simulink model "lab5"  (R2022a)
settings: Solver=ode3  StartTime=0.0  StopTime=Stop_time  FixedStep=1e-6  RelTol=1e-5
undefined symbols (not defined in the file): C_dc_filter, gamma, J_s, k_e, k_m, L_a, R_a, Stop_time, T_e_rated, T_e_st, T_Load, T_sw, tau_m, U_s, U_s_rated
libraries: simulink x13, spsMosfetLib x4, spsCurrentMeasurementLib x3, spsVoltageMeasurementLib x3, spsSeriesRLCBranchLib x2, spsControlledVoltageSourceLib x2, spsDiodeLib x2, spsIGBTLib x1, spspowerguiLib x1
settings Model: Creator=PC  LastModifiedBy=81502
settings SolverCC: ZeroCrossControl=DisableAll  AlgebraicLoopSolver=TrustRegion
settings DataIOCC: LimitDataPoints=on  SaveFormat=Array  SignalLoggingSaveFormat=ModelDataLogs  ReturnWorkspaceOutputs=off
settings OptimizationCC: LifeSpan=inf
settings DebuggingCC: UnderspecifiedInitializationDetection=Classic  MergeDetectMultiDrivingBlocksExec=none  SolverPrmCheckMsg=warning  FcnCallInpInsideContextMsg=warning  UnconnectedInputMsg=warning  UnconnectedOutputMsg=warning  UnconnectedLineMsg=warning  SFUnexpectedBacktrackingDiag=warning  SFNoUnconditionalDefaultTransitionDiag=warning  SFExecutionAtInitializationDiag=none  SFMachineParentedDataDiag=warning  ArithmeticOperatorsInVariantConditions=warning
settings HardwareCC: ProdBitPerPointer=32  ProdBitPerSizeT=32  ProdBitPerPtrDiffT=32  ProdLargestAtomicFloat=None  ProdIntDivRoundTo=Undefined  ProdEndianess=Unspecified  ProdWordSize=32  ProdHWDeviceType=32-bit Generic
settings ModelReferenceCC: PropagateSignalLabelsOutOfModel=off
settings SFSimCC: SimUseLocalCustomCode=off  CustomCodeUndefinedFunction=UseInterfaceOnly
settings RTWCC: RTWUseLocalCustomCode=off  DLArmComputeVersion=19.05
settings CodeAppCC: StateflowObjectComments=on
settings GRTTargetCC: TargetLangStandard=C89/C90 (ANSI)  CombineOutputUpdateFcns=off  GRTInterface=on
settings ConfigComp: CovMetricSettings=dw  CovSaveCumulativeToWorkspaceVar=on  CovSaveSingleToWorkspaceVar=on  CovExternalEMLEnable=off
settings SimscapeCC: SimscapeNormalizeSystem=off

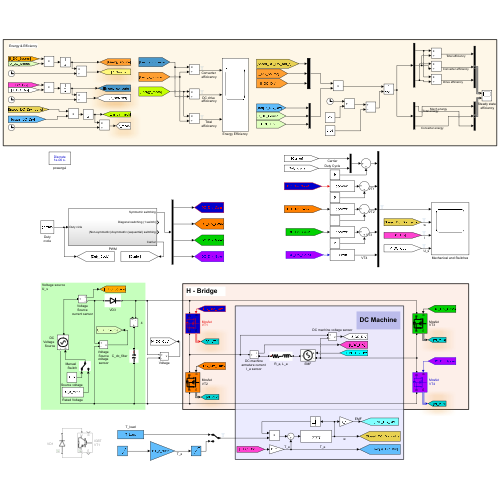
[thumbnail: Simulink's stored preview of the top-level diagram]
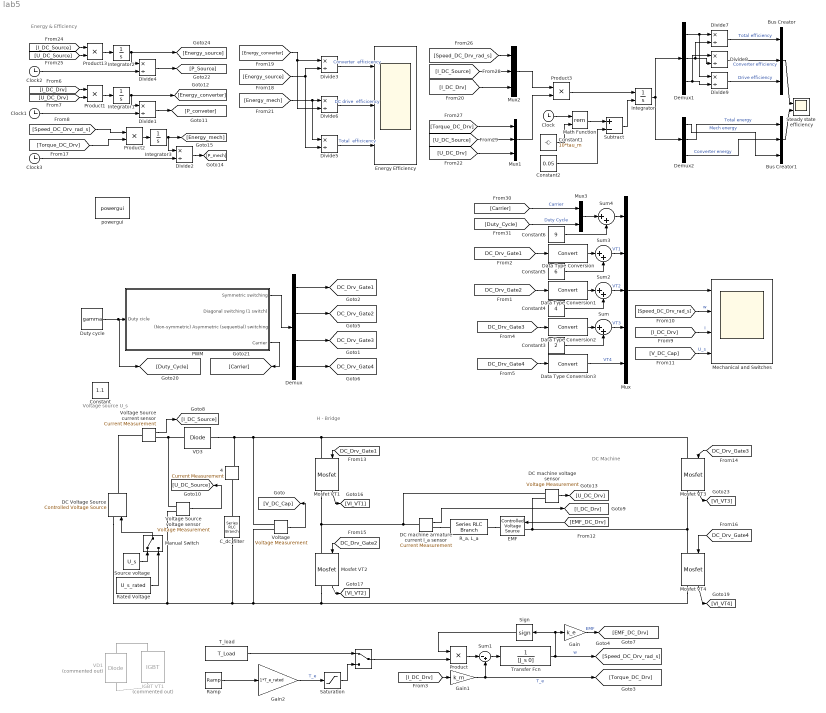
== system lab5 ==
  note: Energy & Efficiency
  note: H - Bridge
  note: Voltage source
      | U_s
  note: DC Machine
  " " : ManualSwitch
  " 4" : spsCurrentMeasurementLib/Current Measurement  PhasorSimulation=off  OutputType=Complex  PSBequivalent=0
  " DC machine armature current I_a sensor" : spsCurrentMeasurementLib/Current Measurement  PhasorSimulation=off  OutputType=Complex  PSBequivalent=0
  " Voltage Source current sensor" : spsCurrentMeasurementLib/Current Measurement  PhasorSimulation=off  OutputType=Complex  PSBequivalent=0
  Bus Creator : BusCreator  Inputs=3
  Bus Creator1 : BusCreator  Inputs=3
  C_dc_filter : spsSeriesRLCBranchLib/Series RLC Branch  LConnTagsString=__new0  RConnTagsString=__new0  BranchType=C  Resistance=0.01  Inductance=1e-2  SetiL0=off  InitialCurrent=0  Capacitance=C_dc_filter  Setx0=on  InitialVoltage=U_s  Measurements=Branch voltage
  Clock{,1..3} (4 alike) : Clock
  Constant1 : Constant  Value=10*tau_m
  Constant2 : Constant  Value=0.05
  Constant3 : Constant  Value=2
  Constant4 : Constant  Value=4
  Constant5 : Constant  Value=6
  Constant6 : Constant  Value=9
  DC Voltage Source : spsControlledVoltageSourceLib/Controlled Voltage Source  Initialize=on  Source_Type=DC  Amplitude=0  Phase=0  Frequency=0  Measurements=None
  DC machine voltage sensor : spsVoltageMeasurementLib/Voltage Measurement  PhasorSimulation=off  OutputType=Complex  PSBequivalent=0
  Data Type Conversion{,1..3} (4 alike) : DataTypeConversion  SaturateOnIntegerOverflow=off  RndMeth=Floor
  Demux : Demux
  Demux1 : Demux  Outputs=3
  Demux2 : Demux  Outputs=3
  Divide{1..9} (9 alike) : Product  Inputs=*/
  Duty cycle : Constant  Value=gamma
  EMF : spsControlledVoltageSourceLib/Controlled Voltage Source  Initialize=on  Source_Type=DC  Amplitude=0  Phase=0  Frequency=0  Measurements=None
  Energy Efficiency : Scope  NumInputPorts=3
  Gain : Gain  Gain=k_e
  Gain1 : Gain  Gain=k_m
  Gain2 : Gain  Gain=1*T_e_rated
  IGBT VT1 : spsIGBTLib/IGBT  Commented=on  Ron=R_on_vt  Lon=0  Vf=Vf_vt  Tf=1e-6  Tt=2e-6  IC=0  Rs=Rs_vt  Cs=Cs_vt  Measurements=on
  Integrator : Integrator  ExternalReset=either
  Integrator1 : Integrator
  Integrator2 : Integrator
  Integrator3 : Integrator
  Manual Switch : ManualSwitch
  Math Function : Math  Operator=rem
  Mechanical and Switches : Scope  NumInputPorts=4
  Mosfet VT{1..4} (4 alike) : spsMosfetLib/Mosfet  Ron=R_on_vt  Lon=0  Rd=R_on_rd  Vfd=Vf_rd  IC=0  Rs=Rs_vt  Cs=Cs_vt  Measurements=on
  Mux : Mux  Inputs=5
  Mux1 : Mux  Inputs=3
  Mux2 : Mux  Inputs=3
  Mux3 : Mux  Inputs=2
  PWM : Subsystem
  Product{,1..3,13} (5 alike) : Product
  "R_a, L_a" : spsSeriesRLCBranchLib/Series RLC Branch  LConnTagsString=__new0  RConnTagsString=__new0  BranchType=RL  Resistance=R_a  Inductance=L_a  SetiL0=off  InitialCurrent=0.1  Capacitance=1e-6  Setx0=off  InitialVoltage=0  Measurements=None
  Ramp : simulink/Sources/Ramp  slope=-T_e_st/T_e_rated/(Stop_time-0.2)  start=0.1  InitialOutput=T_e_st/T_e_rated
  Rated Voltage : Constant  Value=U_s_rated
  Saturation : Saturate  UpperLimit=T_e_st  LowerLimit=-T_e_st
  Sign : Signum
  Source voltage : Constant  Value=U_s
  Steady state efficiency : Scope  NumInputPorts=2
  Subtract : Sum  Inputs=+-
  Sum{,2..4} (4 alike) : Sum  Inputs=|++
  Sum1 : Sum  Inputs=|-+
  T_load : Constant  Value=T_Load
  Transfer Fcn : TransferFcn  Denominator=[J_s 0]
  VD1 : spsDiodeLib/Diode  Commented=on  Ron=R_on_rd  Lon=0  Vf=Vf_rd  IC=0  UseSnubber=off  Rs=inf  Cs=inf  Measurements=off
  VD3 : spsDiodeLib/Diode  Ron=0.00000001  Lon=0  Vf=0.000001  IC=0  UseSnubber=off  Rs=inf  Cs=inf  Measurements=off
  Voltage : spsVoltageMeasurementLib/Voltage Measurement  PhasorSimulation=off  OutputType=Complex  PSBequivalent=0
  Voltage Source voltage sensor : spsVoltageMeasurementLib/Voltage Measurement  PhasorSimulation=off  OutputType=Complex  PSBequivalent=0
  powergui : spspowerguiLib/powergui  Priority=1  SimulationMode=Discrete  SampleTime=1e-6  frequency=60  Iterations=50  frequencyindice=0  Pbase=100e6  ErrMax=1e-4  UnitsV=kV  UnitsW=MW  buscounter=0  FunctionMessages=off  echomessages=off  EnableUseOfTLC=off  CurrentSourceSwitches=off  DisableSnubberDevices=off  DisableRonSwitches=off  DisableVfSwitches=off  DisplayEquations=off  AutomaticDiscreteSolvers=off  SolverType=Tustin/Backward Euler (TBE)  Interpol=off  ExternalGateDelay=off  methode=off  Ts=0  x0status=blocks  SPID=off  SwTol=0  HookPort=off  NonlinearTolerance=1e-4  nMaxIteration=100  ContinueOnMaxIteration=off  RestoreLinks=warning  ResistiveCurrentMeasurement=off  Frange=[0:2:500]  Ylog=off  Xlog=on  ShowGrid=off  save=off  variable=ZData  structure=ScopeData4  ZoomFFT=on  StartTime=0.7  cycles=5  DisplayStyle=3  fundamental=50  FreqAxis=off  MaxFrequency=1000  frequencyindicesteady=1  RmsSteady=1  display=off
  Constant : Constant  IOType=siggen  Value=1.1
  tag scope: DC_Drv_Gate1=global, DC_Drv_Gate2=global, DC_Drv_Gate3=global, DC_Drv_Gate4=global
  wires:
  Sign/1 -> Product/1
  Product/1 -> Sum1/1
  Gain1/1 -> [Torque_DC_Drv], Sum1/2  "T_e"
  Sum1/1 -> Transfer Fcn/1
  Transfer Fcn/1 -> [Speed_DC_Drv_rad_s], Gain/1, Sign/1  "w"
  Gain/1 -> [EMF_DC_Drv]  "EMF"
  [I_DC_Drv] -> Gain1/1
  [DC_Drv_Gate4] -> Mosfet VT4/1
  [EMF_DC_Drv] -> EMF/1
  " DC machine armature current I_a sensor"/1 -> [I_DC_Drv]
  Voltage/1 -> [V_DC_Cap]
  [DC_Drv_Gate2] -> Mosfet VT2/1
  [DC_Drv_Gate1] -> Mosfet VT1/1
  Demux/4 -> [DC_Drv_Gate4]
  Demux/1 -> [DC_Drv_Gate1]
  [DC_Drv_Gate3] -> Mosfet VT3/1
  Integrator2/1 -> Divide4/1, [Energy_source]
  Product13/1 -> Integrator2/1
  [U_DC_Source] -> Product13/2
  Clock2/1 -> Divide4/2
  Divide4/1 -> [P_Source]
  [I_DC_Source] -> Product13/1
  " Voltage Source current sensor"/1 -> [I_DC_Source]
  Voltage Source voltage sensor/1 -> [U_DC_Source]
  [I_DC_Drv] -> Product1/1
  Divide1/1 -> [P_conveter]
  Clock1/1 -> Divide1/2
  [U_DC_Drv] -> Product1/2
  Product1/1 -> Integrator1/1
  Integrator1/1 -> Divide1/1, [Energy_converter]
  DC machine voltage sensor/1 -> [U_DC_Drv]
  Integrator3/1 -> Divide2/1, [Energy_mech]
  Product2/1 -> Integrator3/1
  Clock3/1 -> Divide2/2
  Divide2/1 -> [P_mech]
  [Energy_converter] -> Divide6/2, Divide3/1
  [Energy_source] -> Divide5/2, Divide3/2
  [Energy_mech] -> Divide5/1, Divide6/1
  Divide3/1 -> Energy Efficiency/1  "Converter  efficicency"
  Constant2/1 -> Subtract/2
  Math Function/1 -> Subtract/1
  Subtract/1 -> Integrator/2
  Clock/1 -> Math Function/1
  Constant1/1 -> Math Function/2
  Integrator/1 -> Demux1/1, Demux2/1
  [Speed_DC_Drv_rad_s] -> Product2/1
  [Torque_DC_Drv] -> Product2/2
  Product3/1 -> Integrator/1
  Mux2/1 -> Product3/1
  Mux1/1 -> Product3/2
  [U_DC_Source] -> Mux1/2
  [I_DC_Source] -> Mux2/2
  [Speed_DC_Drv_rad_s] -> Mux2/1
  [Torque_DC_Drv] -> Mux1/1
  Demux/2 -> [DC_Drv_Gate2]
  Constant3/1 -> Sum/2
  Constant4/1 -> Sum2/2
  Constant5/1 -> Sum3/2
  [DC_Drv_Gate4] -> Data Type Conversion3/1
  [DC_Drv_Gate1] -> Data Type Conversion/1
  Data Type Conversion/1 -> Sum3/1
  Data Type Conversion1/1 -> Sum2/1
  Data Type Conversion2/1 -> Sum/1
  Mosfet VT1/1 -> [VI_VT1]
  Mosfet VT2/1 -> [VI_VT2]
  Mosfet VT4/1 -> [VI_VT4]
  Mosfet VT3/1 -> [VI_VT3]
  Manual Switch/1 -> DC Voltage Source/1
  Source voltage/1 -> Manual Switch/1
  Rated Voltage/1 -> Manual Switch/2
  Demux/3 -> [DC_Drv_Gate3]
  Duty cycle/1 -> [Duty_Cycle], PWM/1(Duty cicle)
  [DC_Drv_Gate2] -> Data Type Conversion1/1
  [DC_Drv_Gate3] -> Data Type Conversion2/1
  Mux/1 -> Mechanical and Switches/1
  [Speed_DC_Drv_rad_s] -> Mechanical and Switches/2  "w"
  [V_DC_Cap] -> Mechanical and Switches/4  "U_s"
  [I_DC_Drv] -> Mechanical and Switches/3  "I"
  Ramp/1 -> Gain2/1
  Gain2/1 -> Saturation/1  "T_e"
  Sum3/1 -> Mux/2  "VT1"
  Sum2/1 -> Mux/3  "VT2"
  Sum/1 -> Mux/4  "VT3"
  Data Type Conversion3/1 -> Mux/5  "VT4"
  PWM/4(Carrier) -> [Carrier]
  [Carrier] -> Mux3/1  "Carrier"
  [Duty_Cycle] -> Mux3/2  "Duty Cycle"
  Mux3/1 -> Sum4/1
  Sum4/1 -> Mux/1
  Constant6/1 -> Sum4/2
  Saturation/1 -> " "/2
  T_load/1 -> " "/1
  " "/1 -> Product/2
  Divide6/1 -> Energy Efficiency/2  "DC drive  efficicency"
  Divide5/1 -> Energy Efficiency/3  "Total  efficicency"
  [U_DC_Drv] -> Mux1/3
  [I_DC_Drv] -> Mux2/3
  Demux1/1 -> Divide7/1, Divide9/1
  Demux1/2 -> Divide8/2, Divide7/2
  Demux1/3 -> Divide9/2, Divide8/1
  Divide7/1 -> Bus Creator/1  "Total efficiency"
  Divide8/1 -> Bus Creator/2  "Converter efficiency"
  Divide9/1 -> Bus Creator/3  "Drive efficiency"
  Bus Creator/1 -> Steady state efficiency/1
  Demux2/2 -> Bus Creator1/1  "Total energy"
  Demux2/3 -> Bus Creator1/2  "Converter energy"
  Demux2/1 -> Bus Creator1/3  "Mech energy"
  Bus Creator1/1 -> Steady state efficiency/2
  PWM/1(Symmetric switching) -> Demux/1
  connections:
  C_dc_filter/RConn1 -- Mosfet VT4/RConn1 -- Mosfet VT2/RConn1 -- Voltage/LConn2 -- DC Voltage Source/LConn1 -- Voltage Source voltage sensor/LConn2
  Mosfet VT2/LConn1 -- DC machine voltage sensor/LConn1 -- " DC machine armature current I_a sensor"/LConn1 -- Mosfet VT1/RConn1
  DC machine voltage sensor/LConn2 -- Mosfet VT4/LConn1 -- Mosfet VT3/RConn1 -- EMF/LConn1
  " Voltage Source current sensor"/LConn1 -- DC Voltage Source/RConn1
  Voltage Source voltage sensor/LConn1 -- VD3/LConn1 -- " Voltage Source current sensor"/RConn1
  C_dc_filter/LConn1 -- " 4"/LConn1
  VD1/RConn1 -- IGBT VT1/LConn1
  VD1/LConn1 -- IGBT VT1/RConn1
  VD3/RConn1 -- " 4"/RConn1 -- Voltage/LConn1 -- Mosfet VT3/LConn1 -- Mosfet VT1/LConn1
  "R_a, L_a"/RConn1 -- EMF/RConn1
  " DC machine armature current I_a sensor"/RConn1 -- "R_a, L_a"/LConn1

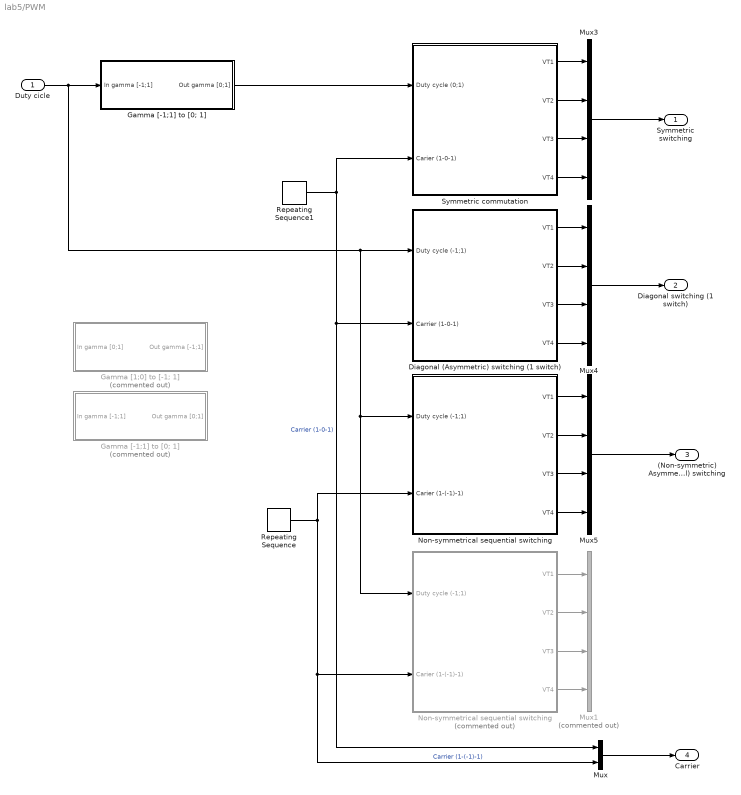
== system lab5/PWM ==
  Duty cicle : Inport
  Diagonal (Asymmetric) switching (1 switch) : Subsystem
  Gamma [-1;1] to [0; 1] : Subsystem  Commented=on
  "Gamma [-1;1] to [0; 1]  " : Subsystem
  Gamma [1;0] to [-1; 1] : Subsystem  Commented=on
  Mux : Mux  Inputs=3
  Mux1 : Mux  Commented=on
  Mux3 : Mux
  Mux4 : Mux
  Mux5 : Mux
  Non-symmetrical sequential switching : Subsystem
  "Non-symmetrical sequential switching  " : Subsystem  Commented=on
  Repeating Sequence : simulink/Sources/Repeating Sequence  rep_seq_t="[0  T_sw/2 T_sw]"  rep_seq_y=[-1 1 -1]
  Repeating Sequence1 : simulink/Sources/Repeating Sequence  rep_seq_t="[0  T_sw/2 T_sw]"  rep_seq_y=[1 0 1]
  "Symmetric commutation " : Subsystem
  Symmetric switching : Outport  VectorParamsAs1DForOutWhenUnconnected=off
  Diagonal switching (1 switch) : Outport  Port=2  VectorParamsAs1DForOutWhenUnconnected=off
  (Non-symmetric) Asymmetric (sequential) switching : Outport  Port=3  VectorParamsAs1DForOutWhenUnconnected=off
  Carrier : Outport  Port=4  VectorParamsAs1DForOutWhenUnconnected=off
  wires:
  Duty cicle/1 -> Diagonal (Asymmetric) switching (1 switch)/1(Duty cycle (-1;1)), "Non-symmetrical sequential switching  "/1(Duty cycle (-1;1)), Non-symmetrical sequential switching/1(Duty cycle (-1;1)), "Gamma [-1;1] to [0; 1]  "/1(In gamma [-1;1])
  "Symmetric commutation "/4(VT4) -> Mux3/4
  "Symmetric commutation "/1(VT1) -> Mux3/1
  "Symmetric commutation "/3(VT3) -> Mux3/3
  "Symmetric commutation "/2(VT2) -> Mux3/2
  Diagonal (Asymmetric) switching (1 switch)/3(VT3) -> Mux4/3
  Diagonal (Asymmetric) switching (1 switch)/4(VT4) -> Mux4/4
  Diagonal (Asymmetric) switching (1 switch)/2(VT2) -> Mux4/2
  Non-symmetrical sequential switching/4(VT4) -> Mux5/4
  Non-symmetrical sequential switching/1(VT1) -> Mux5/1
  Diagonal (Asymmetric) switching (1 switch)/1(VT1) -> Mux4/1
  Mux3/1 -> Symmetric switching/1
  Mux4/1 -> Diagonal switching (1 switch)/1
  Mux5/1 -> (Non-symmetric) Asymmetric (sequential) switching/1
  Non-symmetrical sequential switching/2(VT2) -> Mux5/2
  Non-symmetrical sequential switching/3(VT3) -> Mux5/3
  "Non-symmetrical sequential switching  "/1(VT1) -> Mux1/1
  "Non-symmetrical sequential switching  "/2(VT2) -> Mux1/2
  "Non-symmetrical sequential switching  "/3(VT3) -> Mux1/3
  "Non-symmetrical sequential switching  "/4(VT4) -> Mux1/4
  Repeating Sequence/1 -> "Non-symmetrical sequential switching  "/2(Carier (1-(-1)-1)), Mux/3, Non-symmetrical sequential switching/2(Carier (1-(-1)-1))  "Carrier (1-(-1)-1)"
  Repeating Sequence1/1 -> "Symmetric commutation "/2(Carier (1-0-1)), Mux/1, Diagonal (Asymmetric) switching (1 switch)/2(Carrier (1-0-1))  "Carrier (1-0-1)"
  Mux/1 -> Carrier/1
  "Gamma [-1;1] to [0; 1]  "/1(Out gamma [0;1]) -> "Symmetric commutation "/1(Duty cycle (0;1))

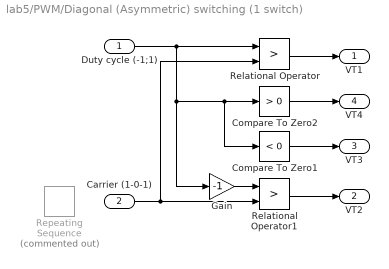
== system lab5/PWM/Diagonal (Asymmetric) switching (1 switch) ==
  Duty cycle (-1;1) : Inport
  Carrier (1-0-1) : Inport  Port=2
  Compare To Zero1 : simulink/Logic and Bit Operations/Compare To Zero  relop=<  OutDataTypeStr=boolean
  Compare To Zero2 : simulink/Logic and Bit Operations/Compare To Zero  relop=>  OutDataTypeStr=boolean
  Gain : Gain  Gain=-1
  Relational Operator : RelationalOperator  Operator=>  OutDataTypeStr=boolean  InputSameDT=off
  Relational Operator1 : RelationalOperator  Operator=>  OutDataTypeStr=boolean  InputSameDT=off
  Repeating Sequence : simulink/Sources/Repeating Sequence  Commented=on  rep_seq_t="[0  T_sw/2 T_sw]"  rep_seq_y=[1 0 1]
  VT1 : Outport  VectorParamsAs1DForOutWhenUnconnected=off
  VT2 : Outport  Port=2  VectorParamsAs1DForOutWhenUnconnected=off
  VT3 : Outport  Port=3  VectorParamsAs1DForOutWhenUnconnected=off
  VT4 : Outport  Port=4  VectorParamsAs1DForOutWhenUnconnected=off
  wires:
  Compare To Zero2/1 -> VT4/1
  Compare To Zero1/1 -> VT3/1
  Duty cycle (-1;1)/1 -> Gain/1, Compare To Zero1/1, Compare To Zero2/1, Relational Operator/1
  Relational Operator/1 -> VT1/1
  Gain/1 -> Relational Operator1/1
  Relational Operator1/1 -> VT2/1
  Carrier (1-0-1)/1 -> Relational Operator1/2, Relational Operator/2

== system lab5/PWM/Gamma [-1;1] to [0; 1] ==
  In gamma [-1;1] : Inport
  Constant1 : Constant
  Gain1 : Gain  Gain=1/2
  Sum1 : Sum  Inputs=|++
  Out gamma [0;1] : Outport
  wires:
  In gamma [-1;1]/1 -> Sum1/1
  Gain1/1 -> Out gamma [0;1]/1
  Sum1/1 -> Gain1/1
  Constant1/1 -> Sum1/2

== system lab5/PWM/Gamma [-1;1] to [0; 1]   ==
  In gamma [-1;1] : Inport
  Constant1 : Constant
  Gain1 : Gain  Gain=1/2
  Sum1 : Sum  Inputs=|++
  Out gamma [0;1] : Outport
  wires:
  Constant1/1 -> Sum1/2
  Sum1/1 -> Gain1/1
  Gain1/1 -> Out gamma [0;1]/1
  In gamma [-1;1]/1 -> Sum1/1

== system lab5/PWM/Gamma [1;0] to [-1; 1] ==
  In gamma [0;1] : Inport
  Constant : Constant
  Gain : Gain  Gain=2
  Sum : Sum  Inputs=|+-
  Out gamma [-1;1] : Outport
  wires:
  Sum/1 -> Out gamma [-1;1]/1
  Constant/1 -> Sum/2
  Gain/1 -> Sum/1
  In gamma [0;1]/1 -> Gain/1

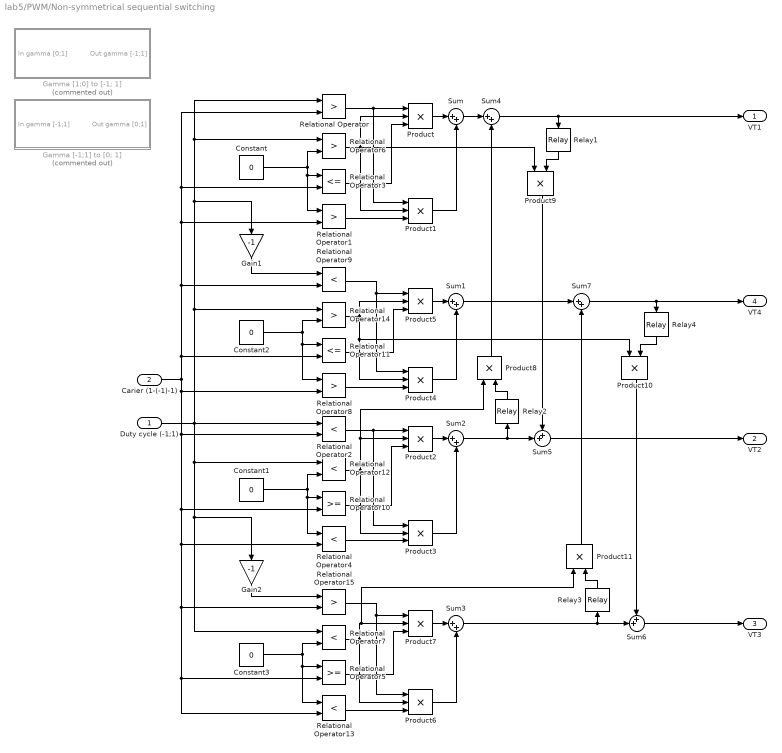
== system lab5/PWM/Non-symmetrical sequential switching ==
  Duty cycle (-1;1) : Inport
  Carier (1-(-1)-1) : Inport  Port=2
  Constant{,1..3} (4 alike) : Constant  Value=0
  Gain1 : Gain  Gain=-1
  Gain2 : Gain  Gain=-1
  Gamma [-1;1] to [0; 1] : Subsystem  Commented=on
  Gamma [1;0] to [-1; 1] : Subsystem  Commented=on
  Product{,1..7} (8 alike) : Product  Inputs=3
  Product{8..11} (4 alike) : Product
  Relational Operator{,1,6,8,14..15} (6 alike) : RelationalOperator  Operator=>  OutDataTypeStr=boolean  InputSameDT=off
  Relational Operator10 : RelationalOperator  OutDataTypeStr=boolean  InputSameDT=off
  Relational Operator11 : RelationalOperator  Operator=<=  OutDataTypeStr=boolean  InputSameDT=off
  Relational Operator{2,4,7,9,12..13} (6 alike) : RelationalOperator  Operator=<  OutDataTypeStr=boolean  InputSameDT=off
  Relational Operator3 : RelationalOperator  Operator=<=  OutDataTypeStr=boolean  InputSameDT=off
  Relational Operator5 : RelationalOperator  OutDataTypeStr=boolean  InputSameDT=off
  Relay{1..4} (4 alike) : Relay  OnSwitchValue=0.999  OffSwitchValue=0.001  OnOutputValue=0  OffOutputValue=1
  Sum{,1..4,7} (6 alike) : Sum  Inputs=|++
  Sum5 : Sum  Inputs=++|
  Sum6 : Sum  Inputs=++|
  VT1 : Outport  VectorParamsAs1DForOutWhenUnconnected=off
  VT2 : Outport  Port=2  VectorParamsAs1DForOutWhenUnconnected=off
  VT3 : Outport  Port=3  VectorParamsAs1DForOutWhenUnconnected=off
  VT4 : Outport  Port=4  VectorParamsAs1DForOutWhenUnconnected=off
  wires:
  Relational Operator10/1 -> Product2/3
  Relational Operator/1 -> Product/1, Product1/1
  Relational Operator3/1 -> Product/3
  Relational Operator9/1 -> Product5/1, Product4/1
  Product4/1 -> Sum1/2
  Constant2/1 -> Relational Operator11/1, Relational Operator8/1, Relational Operator14/2
  Relational Operator14/1 -> Product5/2, Product10/1, Product4/2
  Product1/1 -> Sum/2
  Relational Operator1/1 -> Product1/3
  Constant/1 -> Relational Operator3/1, Relational Operator1/1, Relational Operator6/2
  Relational Operator4/1 -> Product3/3
  Product/1 -> Sum/1
  Product5/1 -> Sum1/1
  Relational Operator8/1 -> Product4/3
  Product7/1 -> Sum3/1
  Constant1/1 -> Relational Operator12/2, Relational Operator4/1, Relational Operator10/1
  Gain2/1 -> Relational Operator15/1
  Relational Operator5/1 -> Product7/3
  Relational Operator2/1 -> Product3/1, Product2/1
  Relational Operator11/1 -> Product5/3
  Sum1/1 -> Sum7/1
  Relational Operator12/1 -> Product3/2, Product2/2, Product8/1
  Relational Operator7/1 -> Product7/2, Product11/1, Product6/2
  Product2/1 -> Sum2/1
  Relational Operator13/1 -> Product6/3
  Product6/1 -> Sum3/2
  Gain1/1 -> Relational Operator9/1
  Relational Operator15/1 -> Product6/1, Product7/1
  Constant3/1 -> Relational Operator7/2, Relational Operator13/1, Relational Operator5/1
  Product3/1 -> Sum2/2
  Sum7/1 -> VT4/1, Relay4/1
  Duty cycle (-1;1)/1 -> Gain1/1, Relational Operator6/1, Relational Operator/1, Relational Operator14/1, Gain2/1, Relational Operator7/1, Relational Operator12/1, Relational Operator2/1
  Sum6/1 -> VT3/1
  Product11/1 -> Sum7/2
  Sum3/1 -> Sum6/2, Relay3/1
  Relay3/1 -> Product11/2
  Product10/1 -> Sum6/1
  Relay4/1 -> Product10/2
  Sum5/1 -> VT2/1
  Sum/1 -> Sum4/1
  Relay2/1 -> Product8/2
  Product9/1 -> Sum5/1
  Product8/1 -> Sum4/2
  Relay1/1 -> Product9/2
  Relational Operator6/1 -> Product1/2, Product9/1, Product/2
  Sum2/1 -> Sum5/2, Relay2/1
  Sum4/1 -> VT1/1, Relay1/1
  Carier (1-(-1)-1)/1 -> Relational Operator11/2, Relational Operator9/2, Relational Operator1/2, Relational Operator3/2, Relational Operator/2, Relational Operator13/2, Relational Operator5/2, Relational Operator15/2, Relational Operator4/2, Relational Operator10/2, Relational Operator2/2, Relational Operator8/2

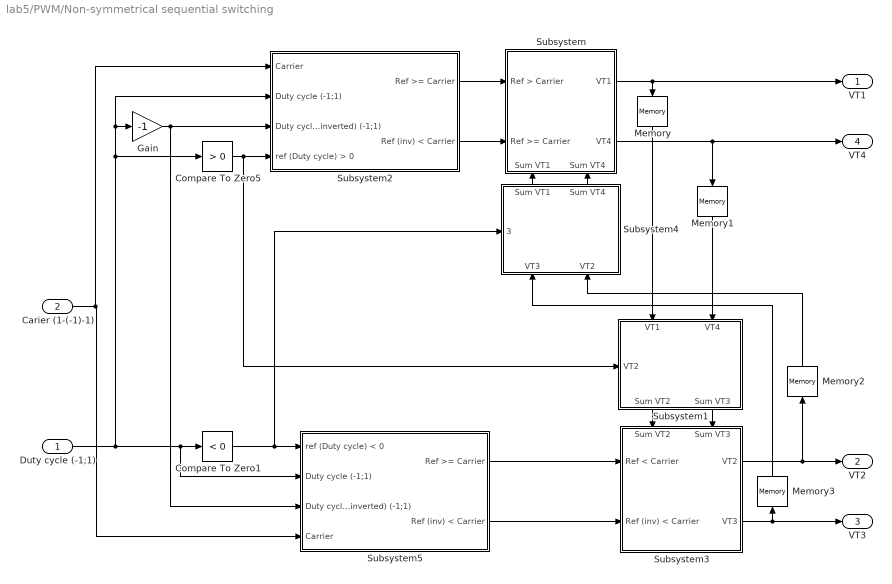
== system lab5/PWM/Non-symmetrical sequential switching   ==
  Duty cycle (-1;1) : Inport
  Carier (1-(-1)-1) : Inport  Port=2
  Compare To Zero1 : simulink/Logic and Bit Operations/Compare To Zero  relop=<  OutDataTypeStr=boolean
  Compare To Zero5 : simulink/Logic and Bit Operations/Compare To Zero  relop=>  OutDataTypeStr=boolean
  Gain : Gain  Gain=-1
  Memory{,1..3} (4 alike) : Memory
  Subsystem : Subsystem
      settings: PortSchema="{\"entries\":[{\"content\":{\"sides\":[{\"content\":{\"connectorIds\":[\"In1\",\"In2\"]},\"type\":\"ConnectorPlacement.EquallySpacedRectSide\",\"uuid\":\"1edc13bd-59e0-4cc0-9bf6-69c0c14bb274\"},{\"content\":{\"connectorIds\":[\"Out1\",\"Out2\"],\"side\":\"RIGHT\"},\"type\":\"ConnectorPlacement.EquallySpacedRectSide\",\"uuid\":\"287b6d5d-6373-4198-a62c-9ab13e508db8\"},{\"content\":{\"connectorIds\":[],\"side\":\"TOP\"},\"type\":\"ConnectorPlacement.EquallySpacedRectSide\",\"uuid\":\"10365a41-7d10-4767-b08d-0380231af0cd\"},{\"content\":{\"connectorIds\":[\"In3\",\"In4\"],\"side\":\"BOTTOM\"},\"type\":\"ConnectorPlacement.EquallySpacedRectSide\",\"uuid\":\"79064c1f-f12c-496a-ad68-e357530a7c3d\"},{\"content\":{\"connectorIds\":[],\"side\":\"HIDDEN\"},\"type\":\"ConnectorPlacement.EquallySpacedRectSide\",\"uuid\":\"c8ec1ad0-0bf0-465f-9247-1d3ffde6369e\"}]},\"type\":\"ConnectorPlacement.EquallySpacedConnector\",\"uuid\":\"859bf412-8161-4eaf-9f32-1e58b98c14d3\"}],\"packageUris\":[\"http://schema.mathworks.com/mf0/Connector/R2020b\"],\"version\":\"1.0\"}"
  Subsystem1 : Subsystem
      settings: PortSchema="{\"entries\":[{\"content\":{\"sides\":[{\"content\":{\"connectorIds\":[\"In1\",\"In2\"]},\"type\":\"ConnectorPlacement.EquallySpacedRectSide\",\"uuid\":\"708c509a-3c1c-41e9-926f-0364c84709fb\"},{\"content\":{\"connectorIds\":[\"Out1\",\"Out2\"],\"side\":\"RIGHT\"},\"type\":\"ConnectorPlacement.EquallySpacedRectSide\",\"uuid\":\"49f51926-54da-4421-ac73-f503aa17b719\"},{\"content\":{\"connectorIds\":[\"In3\"],\"side\":\"TOP\"},\"type\":\"ConnectorPlacement.EquallySpacedRectSide\",\"uuid\":\"75fef89a-0cff-4336-894d-9cbb0e9e9e1a\"},{\"content\":{\"connectorIds\":[],\"side\":\"HIDDEN\"},\"type\":\"ConnectorPlacement.EquallySpacedRectSide\",\"uuid\":\"7c762deb-e236-488c-9487-cd98c1308daa\"}]},\"type\":\"ConnectorPlacement.EquallySpacedConnector\",\"uuid\":\"9fcb198f-e14b-4116-9217-8587d01b960c\"}],\"packageUris\":[\"http://schema.mathworks.com/mf0/Connector/R2020b\"],\"version\":\"1.0\"}"
  Subsystem2 : Subsystem
  Subsystem3 : Subsystem
      settings: PortSchema="{\"entries\":[{\"content\":{\"sides\":[{\"content\":{\"connectorIds\":[\"In1\",\"In2\"]},\"type\":\"ConnectorPlacement.EquallySpacedRectSide\",\"uuid\":\"1edc13bd-59e0-4cc0-9bf6-69c0c14bb274\"},{\"content\":{\"connectorIds\":[\"Out1\",\"Out2\"],\"side\":\"RIGHT\"},\"type\":\"ConnectorPlacement.EquallySpacedRectSide\",\"uuid\":\"287b6d5d-6373-4198-a62c-9ab13e508db8\"},{\"content\":{\"connectorIds\":[\"In3\",\"In4\"],\"side\":\"TOP\"},\"type\":\"ConnectorPlacement.EquallySpacedRectSide\",\"uuid\":\"10365a41-7d10-4767-b08d-0380231af0cd\"},{\"content\":{\"connectorIds\":[],\"side\":\"HIDDEN\"},\"type\":\"ConnectorPlacement.EquallySpacedRectSide\",\"uuid\":\"c8ec1ad0-0bf0-465f-9247-1d3ffde6369e\"}]},\"type\":\"ConnectorPlacement.EquallySpacedConnector\",\"uuid\":\"859bf412-8161-4eaf-9f32-1e58b98c14d3\"}],\"packageUris\":[\"http://schema.mathworks.com/mf0/Connector/R2020b\"],\"version\":\"1.0\"}"
  Subsystem4 : Subsystem
      settings: PortSchema="{\"entries\":[{\"content\":{\"sides\":[{\"content\":{\"connectorIds\":[\"In1\",\"In2\"]},\"type\":\"ConnectorPlacement.EquallySpacedRectSide\",\"uuid\":\"708c509a-3c1c-41e9-926f-0364c84709fb\"},{\"content\":{\"connectorIds\":[\"Out1\",\"Out2\"],\"side\":\"RIGHT\"},\"type\":\"ConnectorPlacement.EquallySpacedRectSide\",\"uuid\":\"49f51926-54da-4421-ac73-f503aa17b719\"},{\"content\":{\"connectorIds\":[\"In3\"],\"side\":\"TOP\"},\"type\":\"ConnectorPlacement.EquallySpacedRectSide\",\"uuid\":\"75fef89a-0cff-4336-894d-9cbb0e9e9e1a\"},{\"content\":{\"connectorIds\":[],\"side\":\"HIDDEN\"},\"type\":\"ConnectorPlacement.EquallySpacedRectSide\",\"uuid\":\"7c762deb-e236-488c-9487-cd98c1308daa\"}]},\"type\":\"ConnectorPlacement.EquallySpacedConnector\",\"uuid\":\"9fcb198f-e14b-4116-9217-8587d01b960c\"}],\"packageUris\":[\"http://schema.mathworks.com/mf0/Connector/R2020b\"],\"version\":\"1.0\"}"
  Subsystem5 : Subsystem
  VT1 : Outport  VectorParamsAs1DForOutWhenUnconnected=off
  VT2 : Outport  Port=2  VectorParamsAs1DForOutWhenUnconnected=off
  VT3 : Outport  Port=3  VectorParamsAs1DForOutWhenUnconnected=off
  VT4 : Outport  Port=4  VectorParamsAs1DForOutWhenUnconnected=off
  wires:
  Subsystem/1(VT1) -> VT1/1, Memory/1
  Compare To Zero5/1 -> Subsystem1/3(VT2), Subsystem2/4(ref (Duty cycle) > 0)
  Subsystem2/1(Ref >= Carrier) -> Subsystem/1(Ref > Carrier)
  Subsystem1/1(Sum VT2) -> Subsystem3/3(Sum VT2)
  Subsystem1/2(Sum VT3) -> Subsystem3/4(Sum VT3)
  Subsystem4/1(Sum VT1) -> Subsystem/3(Sum VT1)
  Subsystem4/2(Sum VT4) -> Subsystem/4(Sum VT4)
  Subsystem3/1(VT2) -> VT2/1, Memory2/1
  Duty cycle (-1;1)/1 -> Subsystem5/2(Duty cycle (-1;1)), Compare To Zero1/1, Subsystem2/2(Duty cycle (-1;1)), Gain/1, Compare To Zero5/1
  Subsystem3/2(VT3) -> VT3/1, Memory3/1
  Memory/1 -> Subsystem1/1(VT1)
  Subsystem/2(VT4) -> VT4/1, Memory1/1
  Memory1/1 -> Subsystem1/2(VT4)
  Memory2/1 -> Subsystem4/2(VT2)
  Memory3/1 -> Subsystem4/1(VT3)
  Subsystem2/2(Ref (inv) < Carrier) -> Subsystem/2(Ref >= Carrier)
  Gain/1 -> Subsystem5/3(Duty cycle (inverted) (-1;1)), Subsystem2/3(Duty cycle (inverted) (-1;1))
  Subsystem5/1(Ref >= Carrier) -> Subsystem3/1(Ref < Carrier)
  Subsystem5/2(Ref (inv) < Carrier) -> Subsystem3/2(Ref (inv) < Carrier)
  Compare To Zero1/1 -> Subsystem4/3(" "), Subsystem5/1(ref (Duty cycle) < 0)
  Carier (1-(-1)-1)/1 -> Subsystem2/1(Carrier), Subsystem5/4(Carrier)

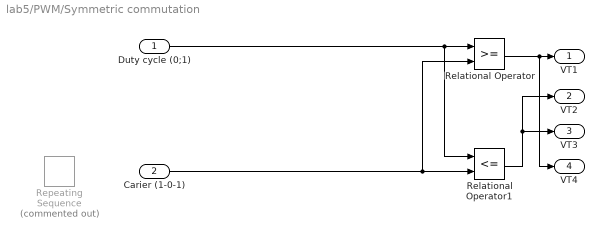
== system lab5/PWM/Symmetric commutation  ==
  Duty cycle (0;1) : Inport
  Carier (1-0-1) : Inport  Port=2
  Relational Operator : RelationalOperator  OutDataTypeStr=boolean  InputSameDT=off
  Relational Operator1 : RelationalOperator  Operator=<=  OutDataTypeStr=boolean  InputSameDT=off
  Repeating Sequence : simulink/Sources/Repeating Sequence  Commented=on  rep_seq_t="[0  T_sw/2 T_sw]"  rep_seq_y=[0 1 0]
  VT1 : Outport  VectorParamsAs1DForOutWhenUnconnected=off
  VT2 : Outport  Port=2  VectorParamsAs1DForOutWhenUnconnected=off
  VT3 : Outport  Port=3  VectorParamsAs1DForOutWhenUnconnected=off
  VT4 : Outport  Port=4  VectorParamsAs1DForOutWhenUnconnected=off
  wires:
  Relational Operator1/1 -> VT2/1, VT3/1
  Relational Operator/1 -> VT1/1, VT4/1
  Duty cycle (0;1)/1 -> Relational Operator1/1, Relational Operator/1
  Carier (1-0-1)/1 -> Relational Operator/2, Relational Operator1/2

== system lab5/PWM/Non-symmetrical sequential switching/Gamma [-1;1] to [0; 1] ==
  In gamma [-1;1] : Inport
  Constant1 : Constant
  Gain1 : Gain  Gain=1/2
  Sum1 : Sum  Inputs=|++
  Out gamma [0;1] : Outport
  wires:
  Constant1/1 -> Sum1/2
  Sum1/1 -> Gain1/1
  Gain1/1 -> Out gamma [0;1]/1
  In gamma [-1;1]/1 -> Sum1/1

== system lab5/PWM/Non-symmetrical sequential switching/Gamma [1;0] to [-1; 1] ==
  In gamma [0;1] : Inport
  Constant : Constant
  Gain : Gain  Gain=2
  Sum : Sum  Inputs=|+-
  Out gamma [-1;1] : Outport
  wires:
  In gamma [0;1]/1 -> Gain/1
  Gain/1 -> Sum/1
  Constant/1 -> Sum/2
  Sum/1 -> Out gamma [-1;1]/1

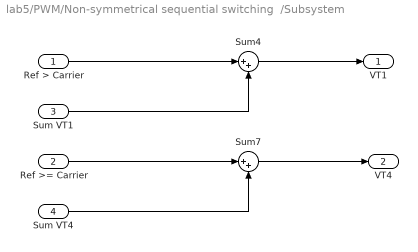
== system lab5/PWM/Non-symmetrical sequential switching  /Subsystem ==
  Ref > Carrier : Inport
  Ref >= Carrier : Inport  Port=2
  Sum VT1 : Inport  Port=3  OutDataTypeStr=uint16
  Sum VT4 : Inport  Port=4  OutDataTypeStr=uint16
  Sum4 : Sum  Inputs=|++
  Sum7 : Sum  Inputs=|++
  VT1 : Outport  OutDataTypeStr=uint16
  VT4 : Outport  Port=2  OutDataTypeStr=uint16
  wires:
  Sum7/1 -> VT4/1
  Sum4/1 -> VT1/1
  Ref > Carrier/1 -> Sum4/1
  Sum VT1/1 -> Sum4/2
  Sum VT4/1 -> Sum7/2
  Ref >= Carrier/1 -> Sum7/1

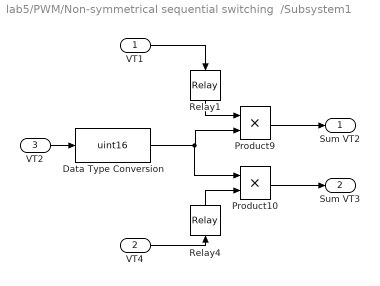
== system lab5/PWM/Non-symmetrical sequential switching  /Subsystem1 ==
  VT1 : Inport
  VT4 : Inport  Port=2
  VT2 : Inport  Port=3
  Data Type Conversion : DataTypeConversion  OutDataTypeStr=uint16  SaturateOnIntegerOverflow=off  RndMeth=Floor
  Product10 : Product  OutDataTypeStr=uint16
  Product9 : Product  OutDataTypeStr=uint16
  Relay1 : Relay  OnSwitchValue=0.999  OffSwitchValue=0.001  OnOutputValue=0  OffOutputValue=1
  Relay4 : Relay  OnSwitchValue=0.999  OffSwitchValue=0.001  OnOutputValue=0  OffOutputValue=1
  Sum VT2 : Outport
  Sum VT3 : Outport  Port=2
  wires:
  Relay1/1 -> Product9/1
  VT4/1 -> Relay4/1
  Relay4/1 -> Product10/2
  VT1/1 -> Relay1/1
  Product9/1 -> Sum VT2/1
  Product10/1 -> Sum VT3/1
  Data Type Conversion/1 -> Product10/1, Product9/2
  VT2/1 -> Data Type Conversion/1

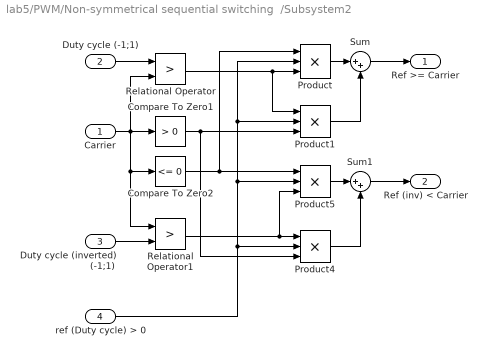
== system lab5/PWM/Non-symmetrical sequential switching  /Subsystem2 ==
  Carrier : Inport
  Duty cycle (-1;1) : Inport  Port=2
  Duty cycle (inverted) (-1;1) : Inport  Port=3
  ref (Duty cycle) > 0 : Inport  Port=4
  Compare To Zero1 : simulink/Logic and Bit Operations/Compare To Zero  relop=>  OutDataTypeStr=boolean
  Compare To Zero2 : simulink/Logic and Bit Operations/Compare To Zero  relop=<=  OutDataTypeStr=boolean
  Product{,1,4..5} (4 alike) : Product  Inputs=3
  Relational Operator : RelationalOperator  Operator=>  OutDataTypeStr=boolean  InputSameDT=off
  Relational Operator1 : RelationalOperator  Operator=>  OutDataTypeStr=boolean  InputSameDT=off
  Sum : Sum  Inputs=|++
  Sum1 : Sum  Inputs=|++
  Ref >= Carrier : Outport
  Ref (inv) < Carrier : Outport  Port=2
  wires:
  Compare To Zero1/1 -> Product4/3, Product1/3
  Carrier/1 -> Relational Operator/2, Compare To Zero1/1, Relational Operator1/1, Compare To Zero2/1
  Compare To Zero2/1 -> Product5/1, Product/1
  Product5/1 -> Sum1/1
  ref (Duty cycle) > 0/1 -> Product/2, Product1/2, Product5/2, Product4/2
  Product4/1 -> Sum1/2
  Product1/1 -> Sum/2
  Sum1/1 -> Ref (inv) < Carrier/1
  Duty cycle (-1;1)/1 -> Relational Operator/1
  Product/1 -> Sum/1
  Sum/1 -> Ref >= Carrier/1
  Relational Operator1/1 -> Product5/3, Product4/1
  Duty cycle (inverted) (-1;1)/1 -> Relational Operator1/2
  Relational Operator/1 -> Product/3, Product1/1

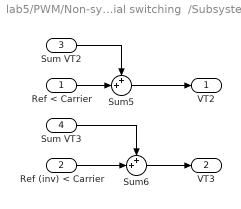
== system lab5/PWM/Non-symmetrical sequential switching  /Subsystem3 ==
  Ref < Carrier : Inport
  Ref (inv) < Carrier : Inport  Port=2
  Sum VT2 : Inport  Port=3
  Sum VT3 : Inport  Port=4
  Sum5 : Sum  Inputs=++|
  Sum6 : Sum  Inputs=++|
  VT2 : Outport  VectorParamsAs1DForOutWhenUnconnected=off
  VT3 : Outport  Port=2  VectorParamsAs1DForOutWhenUnconnected=off
  wires:
  Ref < Carrier/1 -> Sum5/2
  Ref (inv) < Carrier/1 -> Sum6/2
  Sum6/1 -> VT3/1
  Sum VT2/1 -> Sum5/1
  Sum5/1 -> VT2/1
  Sum VT3/1 -> Sum6/1

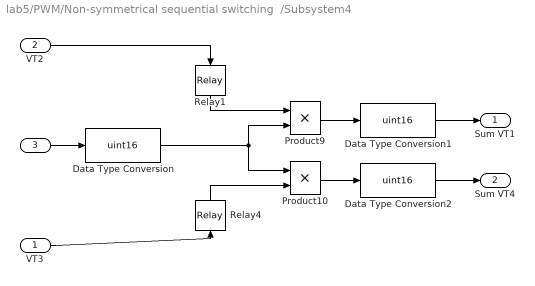
== system lab5/PWM/Non-symmetrical sequential switching  /Subsystem4 ==
  VT3 : Inport
  VT2 : Inport  Port=2
  " " : Inport  Port=3
  Data Type Conversion : DataTypeConversion  OutDataTypeStr=uint16  SaturateOnIntegerOverflow=off  RndMeth=Floor
  Data Type Conversion1 : DataTypeConversion  OutDataTypeStr=uint16  SaturateOnIntegerOverflow=off  RndMeth=Floor
  Data Type Conversion2 : DataTypeConversion  OutDataTypeStr=uint16  SaturateOnIntegerOverflow=off  RndMeth=Floor
  Product10 : Product  OutDataTypeStr=uint32
  Product9 : Product  OutDataTypeStr=uint32
  Relay1 : Relay  OnSwitchValue=0.999  OffSwitchValue=0.001  OnOutputValue=0  OffOutputValue=1
  Relay4 : Relay  OnSwitchValue=0.999  OffSwitchValue=0.001  OnOutputValue=0  OffOutputValue=1
  Sum VT1 : Outport
  Sum VT4 : Outport  Port=2
  wires:
  Product10/1 -> Data Type Conversion2/1
  Product9/1 -> Data Type Conversion1/1
  VT2/1 -> Relay1/1
  Relay4/1 -> Product10/2
  VT3/1 -> Relay4/1
  Relay1/1 -> Product9/1
  Data Type Conversion/1 -> Product10/1, Product9/2
  Data Type Conversion1/1 -> Sum VT1/1
  Data Type Conversion2/1 -> Sum VT4/1
  " "/1 -> Data Type Conversion/1

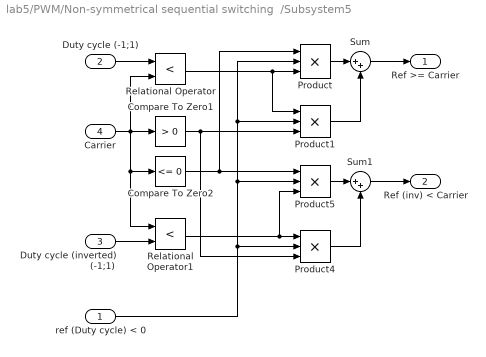
== system lab5/PWM/Non-symmetrical sequential switching  /Subsystem5 ==
  ref (Duty cycle) < 0 : Inport
  Duty cycle (-1;1) : Inport  Port=2
  Duty cycle (inverted) (-1;1) : Inport  Port=3
  Carrier : Inport  Port=4
  Compare To Zero1 : simulink/Logic and Bit Operations/Compare To Zero  relop=>  OutDataTypeStr=boolean
  Compare To Zero2 : simulink/Logic and Bit Operations/Compare To Zero  relop=<=  OutDataTypeStr=boolean
  Product{,1,4..5} (4 alike) : Product  Inputs=3
  Relational Operator : RelationalOperator  Operator=<  OutDataTypeStr=boolean  InputSameDT=off
  Relational Operator1 : RelationalOperator  Operator=<  OutDataTypeStr=boolean  InputSameDT=off
  Sum : Sum  Inputs=|++
  Sum1 : Sum  Inputs=|++
  Ref >= Carrier : Outport
  Ref (inv) < Carrier : Outport  Port=2
  wires:
  Relational Operator/1 -> Product1/1, Product/3
  Duty cycle (inverted) (-1;1)/1 -> Relational Operator1/2
  Relational Operator1/1 -> Product4/1, Product5/3
  Sum/1 -> Ref >= Carrier/1
  Product/1 -> Sum/1
  Duty cycle (-1;1)/1 -> Relational Operator/1
  Sum1/1 -> Ref (inv) < Carrier/1
  Product1/1 -> Sum/2
  Product4/1 -> Sum1/2
  ref (Duty cycle) < 0/1 -> Product4/2, Product5/2, Product1/2, Product/2
  Product5/1 -> Sum1/1
  Compare To Zero2/1 -> Product/1, Product5/1
  Carrier/1 -> Compare To Zero2/1, Relational Operator1/1, Compare To Zero1/1, Relational Operator/2
  Compare To Zero1/1 -> Product1/3, Product4/3
